simulink model "scattering_FP"  (R2021b)
settings: Solver=ode45  StartTime=0.0  StopTime=25  FixedStep=Ts  MinStep=1e-5  RelTol=1e-5
undefined symbols (not defined in the file): A, A_int, B, b, Be, Bh_i, Bs, C, delayT, Dh, DiscIntNeverNeededParam, Discrete, Dm, Ds, Fc, Ff, Fip, forceNoiseVariance, Jh_i, Ke, Kh, Kh_i, Ks, Mm, Ms, posNoiseVariance, R, Time, Ts, x0, xe
libraries: simulink x3, ctrlSharedLib x2, cstblocks x1
settings Model: Creator=simon  LastModifiedBy=miche
settings SolverCC: AlgebraicLoopSolver=LineSearch
settings DebuggingCC: SFMachineParentedDataDiag=warning

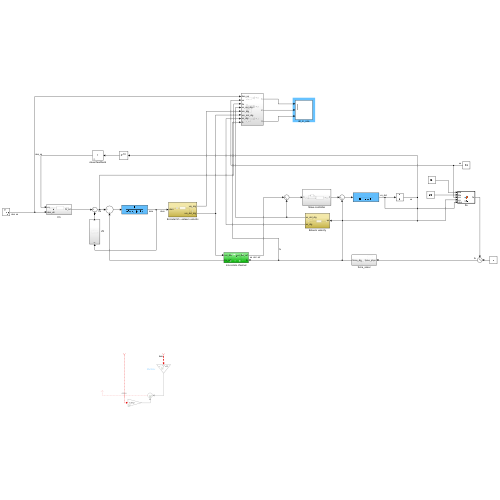
[thumbnail: Simulink's stored preview of the top-level diagram]
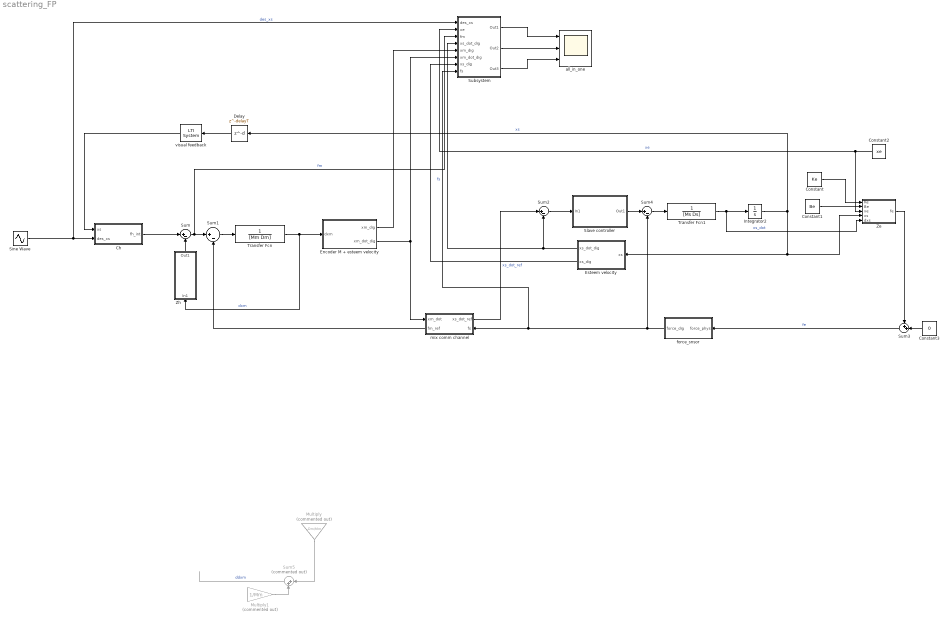
== system scattering_FP ==
  Ch : Subsystem
  Constant : Constant  Value=Ke
  Constant1 : Constant  Value=Be
  Constant2 : Constant  Value=xe
  Constant3 : Constant  Value=0
  Delay : Delay  DelayLength=delayT
  Encoder M + esteem velocity : Subsystem
  Esteem velocity : Subsystem
  Integrator2 : Integrator
  Multiply : Gain  Commented=on  Gain=-Dm/Mm
  Multiply1 : Gain  Commented=on  Gain=1/Mm
  Sine Wave : Sin  Amplitude=A_int  Frequency=Fc  SampleTime=0
  Slave controller : Subsystem
  Subsystem : Subsystem
  Sum{,1..2,4} (4 alike) : Sum  Inputs=|+-
  Sum3 : Sum  Inputs=++|
  Sum5 : Sum  Commented=on  Inputs=|++
  Transfer Fcn : TransferFcn  Denominator=[Mm Dm]
  Transfer Fcn1 : TransferFcn  Denominator=[Ms Ds]
  Ze : MATLAB Function  TreatAsAtomicUnit=on
  Zh : Subsystem
  all_in_one : Scope  NumInputPorts=3
  force_snsor : Subsystem
  mix comm channel : Subsystem
      settings: PortSchema="{\"entries\":[{\"content\":{\"sides\":[{\"content\":{\"connectorIds\":[\"In1\",\"Out2\"]},\"type\":\"ConnectorPlacement.EquallySpacedRectSide\",\"uuid\":\"b52b5263-ec77-4a5b-a444-fedf8384a1f4\"},{\"content\":{\"connectorIds\":[\"Out1\",\"In2\"],\"side\":\"RIGHT\"},\"type\":\"ConnectorPlacement.EquallySpacedRectSide\",\"uuid\":\"29fc6d0d-53a2-4de5-b8fc-fdc6e2130f9a\"},{\"content\":{\"connectorIds\":[],\"side\":\"TOP\"},\"type\":\"ConnectorPlacement.EquallySpacedRectSide\",\"uuid\":\"d00abe1a-0b08-4fbd-831b-b235aed68611\"},{\"content\":{\"connectorIds\":[],\"side\":\"HIDDEN\"},\"type\":\"ConnectorPlacement.EquallySpacedRectSide\",\"uuid\":\"d0d3daa3-ebbf-4bb5-b3d9-7ef522d44ef5\"}]},\"type\":\"ConnectorPlacement.EquallySpacedConnector\",\"uuid\":\"e5a03f62-d534-4700-82c8-2ace6ee2abeb\"}],\"packageUris\":[\"http://schema.mathworks.com/mf0/Connector/R2020b\"],\"version\":\"1.0\"}"
  visual feedback : cstblocks/LTI System  sys=1  IC=[]
  wires:
  Zh/1(Out1) -> Sum/2
  Sum4/1 -> Transfer Fcn1/1
  Transfer Fcn1/1 -> Ze/5(dxs), Integrator2/1  "xs_dot"
  Ze/1(fe) -> Sum3/1
  Integrator2/1 -> Esteem velocity/1(xs), Ze/4(xs), Delay/1  "xs"
  Constant2/1 -> Ze/3(xe), Subsystem/2(xe)  "xe"
  Constant1/1 -> Ze/2(Be)
  Constant/1 -> Ze/1(Ke)
  Sum/1 -> Subsystem/3(fm), Sum1/1  "fm"
  Transfer Fcn/1 -> Zh/1(In1), Encoder M + esteem velocity/1(dxm)  "dxm"
  mix comm channel/2(fm_ref) -> Sum1/2
  mix comm channel/1(xs_dot_ref) -> Sum2/1  "xs_dot_ref"
  Sum3/1 -> force_snsor/1(force_phys)  "fe"
  Constant3/1 -> Sum3/2
  Ch/1(fh_int) -> Sum/1
  visual feedback/1 -> Ch/1(xs)
  force_snsor/1(force_dig) -> Sum4/2, Subsystem/8(fs), mix comm channel/2(fs)  "fs"
  Sine Wave/1 -> Subsystem/1(des_xs), Ch/2(des_xs)  "des_xs"
  Sum1/1 -> Transfer Fcn/1
  Delay/1 -> visual feedback/1
  ? -> Multiply1/1
  Sum5/1 -> ?  "ddxm"
  Multiply/1 -> Sum5/1
  ? -> Multiply/1  "dxm"
  Multiply1/1 -> Sum5/2
  Encoder M + esteem velocity/2(xm_dot_dig) -> mix comm channel/1(xm_dot), Subsystem/6(xm_dot_dig)
  Esteem velocity/1(xs_dot_dig) -> Sum2/2, Subsystem/4(xs_dot_dig)
  Sum2/1 -> Slave controller/1(In1)
  Slave controller/1(Out1) -> Sum4/1
  Encoder M + esteem velocity/1(xm_dig) -> Subsystem/5(xm_dig)
  Esteem velocity/2(xs_dig) -> Subsystem/7(xs_dig)
  Subsystem/1(Out1) -> all_in_one/1
  Subsystem/2(Out2) -> all_in_one/2
  Subsystem/3(Out3) -> all_in_one/3

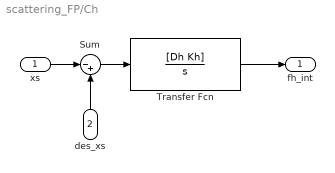
== system scattering_FP/Ch ==
  xs : Inport
  des_xs : Inport  Port=2
  Sum : Sum  Inputs=|-+
  Transfer Fcn : TransferFcn  Numerator=[Dh Kh]  Denominator=[1 0]
  fh_int : Outport
  wires:
  xs/1 -> Sum/1
  des_xs/1 -> Sum/2
  Sum/1 -> Transfer Fcn/1
  Transfer Fcn/1 -> fh_int/1

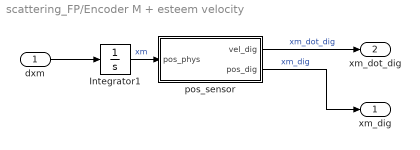
== system scattering_FP/Encoder M + esteem velocity ==
  dxm : Inport
  Integrator1 : Integrator
  pos_sensor : Subsystem
  xm_dig : Outport
  xm_dot_dig : Outport  Port=2
  wires:
  Integrator1/1 -> pos_sensor/1(pos_phys)  "xm"
  pos_sensor/1(vel_dig) -> xm_dot_dig/1  "xm_dot_dig"
  dxm/1 -> Integrator1/1
  pos_sensor/2(pos_dig) -> xm_dig/1  "xm_dig"

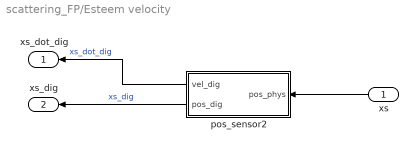
== system scattering_FP/Esteem velocity ==
  xs : Inport
  pos_sensor2 : Subsystem
  xs_dot_dig : Outport
  xs_dig : Outport  Port=2
  wires:
  pos_sensor2/2(pos_dig) -> xs_dig/1  "xs_dig"
  xs/1 -> pos_sensor2/1(pos_phys)
  pos_sensor2/1(vel_dig) -> xs_dot_dig/1  "xs_dot_dig"

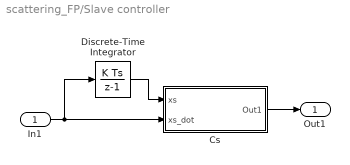
== system scattering_FP/Slave controller ==
  In1 : Inport
  Cs : Subsystem
  Discrete-Time Integrator : DiscreteIntegrator  SampleTime=-1  ICPrevOutput=DiscIntNeverNeededParam  ICPrevScaledInput=DiscIntNeverNeededParam
  Out1 : Outport
  wires:
  In1/1 -> Cs/2(xs_dot), Discrete-Time Integrator/1
  Discrete-Time Integrator/1 -> Cs/1(xs)
  Cs/1(Out1) -> Out1/1

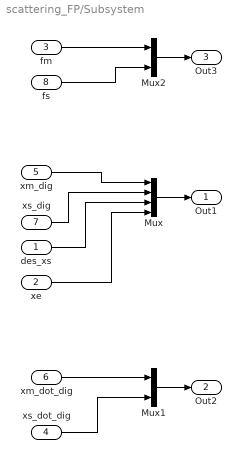
== system scattering_FP/Subsystem ==
  des_xs : Inport
  xe : Inport  Port=2
  fm : Inport  Port=3
  xs_dot_dig : Inport  Port=4
  xm_dig : Inport  Port=5
  xm_dot_dig : Inport  Port=6
  xs_dig : Inport  Port=7
  fs : Inport  Port=8
  Mux : Mux
  Mux1 : Mux  Inputs=2
  Mux2 : Mux  Inputs=2
  Out1 : Outport
  Out2 : Outport  Port=2
  Out3 : Outport  Port=3
  wires:
  Mux1/1 -> Out2/1
  xe/1 -> Mux/4
  xm_dot_dig/1 -> Mux1/1
  Mux2/1 -> Out3/1
  xm_dig/1 -> Mux/1
  xs_dig/1 -> Mux/2
  fs/1 -> Mux2/2
  fm/1 -> Mux2/1
  xs_dot_dig/1 -> Mux1/2
  Mux/1 -> Out1/1
  des_xs/1 -> Mux/3

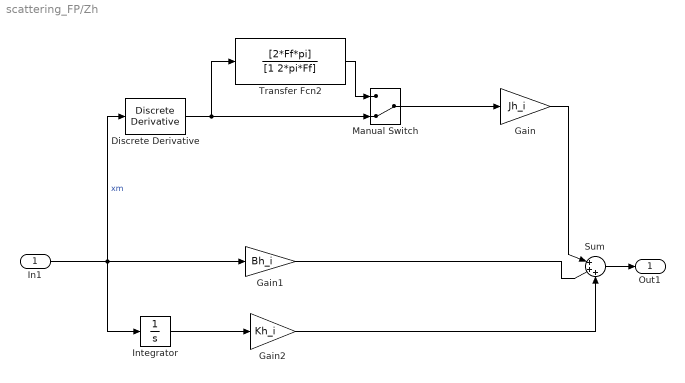
== system scattering_FP/Zh ==
  In1 : Inport
  Discrete Derivative : simulink/Discrete/Discrete Derivative  gainval=1.0  ICPrevScaledInput=0.0  OutMin=[]  OutMax=[]  OutDataType=fixdt(1, 16)  OutScaling=2^-10  DoSatur=off
  Gain : Gain  Gain=Jh_i
  Gain1 : Gain  Gain=Bh_i
  Gain2 : Gain  Gain=Kh_i
  Integrator : Integrator
  Manual Switch : ManualSwitch  CurrentSetting=0
  Sum : Sum  Inputs=|+++
  Transfer Fcn2 : TransferFcn  Numerator=[2*Ff*pi]  Denominator=[1 2*pi*Ff]
  Out1 : Outport
  wires:
  Gain/1 -> Sum/1
  Gain1/1 -> Sum/2
  Gain2/1 -> Sum/3
  Sum/1 -> Out1/1
  In1/1 -> Integrator/1, Gain1/1, Discrete Derivative/1  "xm"
  Integrator/1 -> Gain2/1
  Manual Switch/1 -> Gain/1
  Discrete Derivative/1 -> Transfer Fcn2/1, Manual Switch/2
  Transfer Fcn2/1 -> Manual Switch/1

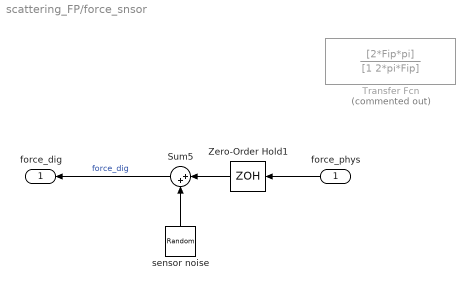
== system scattering_FP/force_snsor ==
  force_phys : Inport
  Sum5 : Sum  Inputs=|++
  Transfer Fcn : TransferFcn  Commented=on  Numerator=[2*Fip*pi]  Denominator=[1 2*pi*Fip]
  Zero-Order Hold1 : ZeroOrderHold  SampleTime=Ts
  sensor noise : RandomNumber  Variance=forceNoiseVariance  SampleTime=Ts
  force_dig : Outport
  wires:
  Sum5/1 -> force_dig/1  "force_dig"
  Zero-Order Hold1/1 -> Sum5/1
  sensor noise/1 -> Sum5/2
  force_phys/1 -> Zero-Order Hold1/1

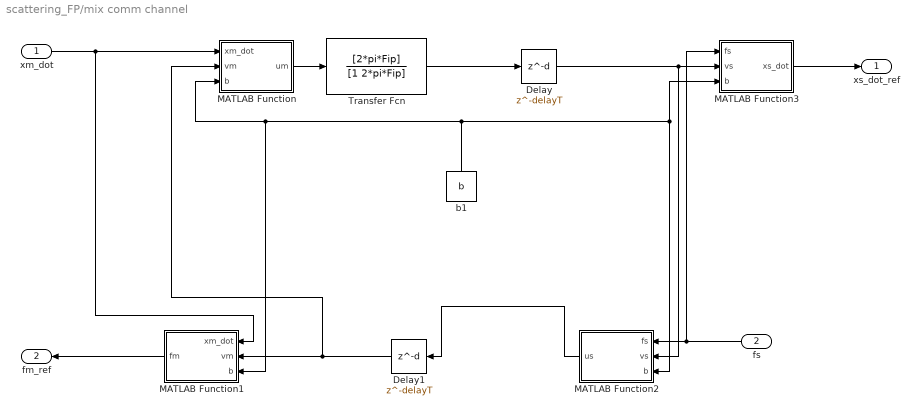
== system scattering_FP/mix comm channel ==
  xm_dot : Inport
  fs : Inport  Port=2
  Delay : Delay  DelayLength=delayT  SampleTime=Ts
  Delay1 : Delay  DelayLength=delayT  SampleTime=Ts
  MATLAB Function : MATLAB Function  TreatAsAtomicUnit=on
  MATLAB Function1 : MATLAB Function  TreatAsAtomicUnit=on
  MATLAB Function2 : MATLAB Function  TreatAsAtomicUnit=on
  MATLAB Function3 : MATLAB Function  TreatAsAtomicUnit=on
  Transfer Fcn : TransferFcn  Numerator=[2*pi*Fip]  Denominator=[1 2*pi*Fip]
  b1 : Constant  Value=b
  xs_dot_ref : Outport
  fm_ref : Outport  Port=2
  wires:
  b1/1 -> MATLAB Function2/3(b), MATLAB Function3/3(b), MATLAB Function1/3(b), MATLAB Function/3(b)
  xm_dot/1 -> MATLAB Function1/1(xm_dot), MATLAB Function/1(xm_dot)
  MATLAB Function1/1(fm) -> fm_ref/1
  fs/1 -> MATLAB Function3/1(fs), MATLAB Function2/1(fs)
  MATLAB Function3/1(xs_dot) -> xs_dot_ref/1
  MATLAB Function/1(um) -> Transfer Fcn/1
  Delay/1 -> MATLAB Function2/2(vs), MATLAB Function3/2(vs)
  Delay1/1 -> MATLAB Function/2(vm), MATLAB Function1/2(vm)
  Transfer Fcn/1 -> Delay/1
  MATLAB Function2/1(us) -> Delay1/1

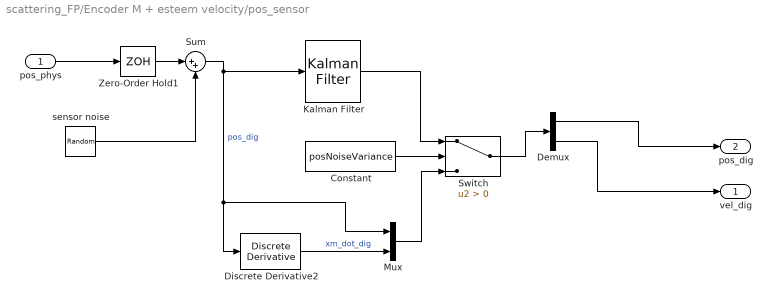
== system scattering_FP/Encoder M + esteem velocity/pos_sensor ==
  pos_phys : Inport
  Constant : Constant  Value=posNoiseVariance
  Demux : Demux  Outputs=2
  Discrete Derivative2 : simulink/Discrete/Discrete Derivative  gainval=1.0  ICPrevScaledInput=0.0  OutMin=[]  OutMax=[]  OutDataType=fixdt(1, 16)  OutScaling=2^-10  DoSatur=off
  Kalman Filter : ctrlSharedLib/Kalman Filter  TimeDomain=Discrete-Time  UseCurrentEstimator=on  ModelSource=Individual A, B, C, D matrices  ModelSourceVariable=ss(0.95,1,1,0,1)  A=A  B=B  C=C  D=0  NumberOfStates=2  NumberOfInputs=1  NumberOfOutputs=1  InitialEstimateSource=Dialog  X0=x0  P0=10  UseK=off  UseGH=off  NumberOfProcessNoiseInputs=1  G=1  TimeInvariantG=on  H=0  TimeInvariantH=on  Q=Q_m  TimeInvariantQ=on  R=R  TimeInvariantR=on  N=0  TimeInvariantN=on  AddInputPort=off  AddEnablePort=off  OutputEstimatedY=off  OutputP=off  Ts=Ts
  Mux : Mux  Inputs=2
  Sum : Sum  Inputs=|++
  Switch : Switch  Criteria=u2 > Threshold
  Zero-Order Hold1 : ZeroOrderHold  SampleTime=Ts
  sensor noise : RandomNumber  Variance=posNoiseVariance  SampleTime=Ts
  vel_dig : Outport
  pos_dig : Outport  Port=2
  wires:
  pos_phys/1 -> Zero-Order Hold1/1
  Zero-Order Hold1/1 -> Sum/1
  sensor noise/1 -> Sum/2
  Kalman Filter/1 -> Switch/1
  Sum/1 -> Mux/1, Discrete Derivative2/1, Kalman Filter/1  "pos_dig"
  Constant/1 -> Switch/2
  Mux/1 -> Switch/3
  Discrete Derivative2/1 -> Mux/2  "xm_dot_dig"
  Switch/1 -> Demux/1
  Demux/1 -> pos_dig/1
  Demux/2 -> vel_dig/1

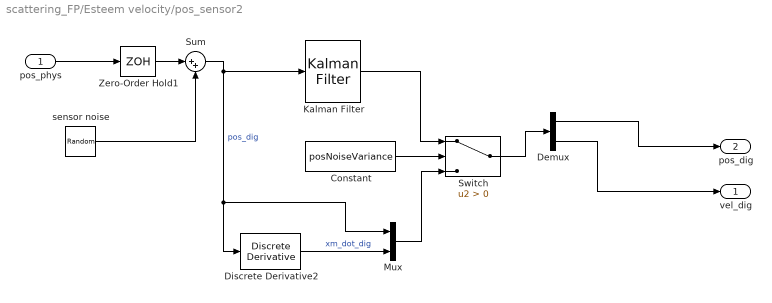
== system scattering_FP/Esteem velocity/pos_sensor2 ==
  pos_phys : Inport
  Constant : Constant  Value=posNoiseVariance
  Demux : Demux  Outputs=2
  Discrete Derivative2 : simulink/Discrete/Discrete Derivative  gainval=1.0  ICPrevScaledInput=0.0  OutMin=[]  OutMax=[]  OutDataType=fixdt(1, 16)  OutScaling=2^-10  DoSatur=off
  Kalman Filter : ctrlSharedLib/Kalman Filter  TimeDomain=Discrete-Time  UseCurrentEstimator=on  ModelSource=Individual A, B, C, D matrices  ModelSourceVariable=ss(0.95,1,1,0,1)  A=A  B=B  C=C  D=0  NumberOfStates=2  NumberOfInputs=1  NumberOfOutputs=1  InitialEstimateSource=Dialog  X0=0  P0=10  UseK=off  UseGH=off  NumberOfProcessNoiseInputs=1  G=1  TimeInvariantG=on  H=0  TimeInvariantH=on  Q=Q_m  TimeInvariantQ=on  R=R  TimeInvariantR=on  N=0  TimeInvariantN=on  AddInputPort=off  AddEnablePort=off  OutputEstimatedY=off  OutputP=off  Ts=Ts
  Mux : Mux  Inputs=2
  Sum : Sum  Inputs=|++
  Switch : Switch  Criteria=u2 > Threshold
  Zero-Order Hold1 : ZeroOrderHold  SampleTime=Ts
  sensor noise : RandomNumber  Variance=posNoiseVariance  SampleTime=Ts
  vel_dig : Outport
  pos_dig : Outport  Port=2
  wires:
  pos_phys/1 -> Zero-Order Hold1/1
  Zero-Order Hold1/1 -> Sum/1
  sensor noise/1 -> Sum/2
  Kalman Filter/1 -> Switch/1
  Sum/1 -> Mux/1, Discrete Derivative2/1, Kalman Filter/1  "pos_dig"
  Constant/1 -> Switch/2
  Mux/1 -> Switch/3
  Discrete Derivative2/1 -> Mux/2  "xm_dot_dig"
  Switch/1 -> Demux/1
  Demux/1 -> pos_dig/1
  Demux/2 -> vel_dig/1

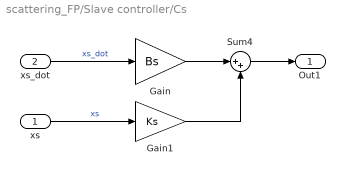
== system scattering_FP/Slave controller/Cs ==
  xs : Inport
  xs_dot : Inport  Port=2
  Gain : Gain  Gain=Bs
  Gain1 : Gain  Gain=Ks
  Sum4 : Sum  Inputs=|++
  Out1 : Outport
  wires:
  Gain1/1 -> Sum4/2
  Sum4/1 -> Out1/1
  xs_dot/1 -> Gain/1  "xs_dot"
  Gain/1 -> Sum4/1
  xs/1 -> Gain1/1  "xs"

== matlab function scattering_FP/Ze ==
  data: Ke input; fe output; Be input; xe input; xs input; dxs input
function fe = env(Ke, Be, xe, xs, dxs)
    if xs > xe
        fe = Ke*(xs-xe)+Be*max(dxs, 0);
    else
        fe = 0;
    end

== matlab function scattering_FP/mix comm channel/MATLAB Function ==
  data: xm_dot input; um output; vm input; b input
function um = fcn(xm_dot, vm, b)

um = sqrt(2*b)*xm_dot+vm;

== matlab function scattering_FP/mix comm channel/MATLAB Function1 ==
  data: xm_dot input; fm output; vm input; b input
function fm = fcn(xm_dot, vm, b)

fm = b*xm_dot+sqrt(2*b)*vm;

== matlab function scattering_FP/mix comm channel/MATLAB Function2 ==
  data: fs input; us output; vs input; b input
function us = fcn(fs, vs, b)

us = sqrt(2/b)*fs-vs;

== matlab function scattering_FP/mix comm channel/MATLAB Function3 ==
  data: fs input; xs_dot output; vs input; b input
function xs_dot = fcn(fs, vs, b)

xs_dot = -1/b*(fs-sqrt(2*b)*vs);
